simulink subsystem "Trayectoria"  (R2024b)
settings: Solver=VariableStepAuto  StartTime=0.0  StopTime=10.0  RelTol=1e-3
libraries: slpidlib x1
settings Model: Creator=Chenfu  LastModifiedBy=Chenfu

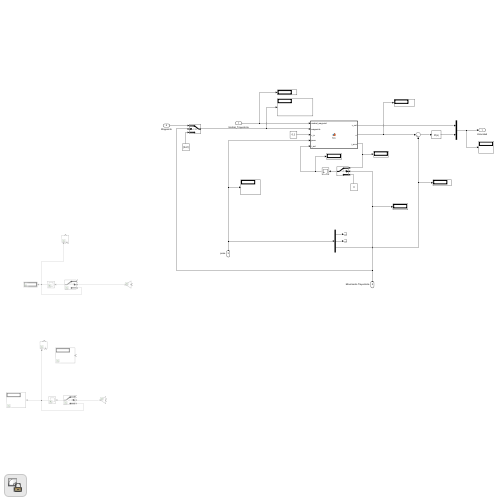
[thumbnail: Simulink's stored preview of the top-level diagram]
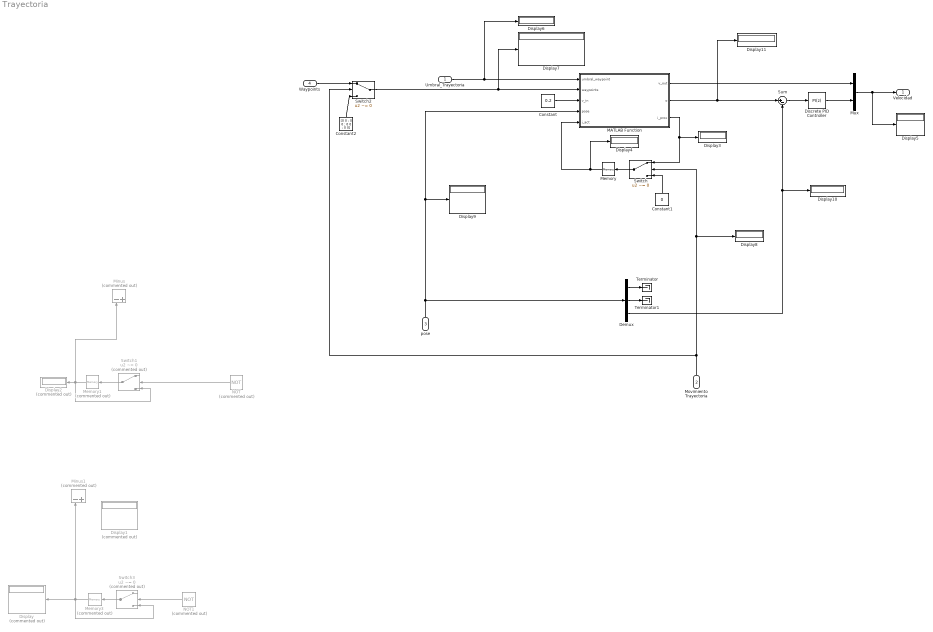
== system Trayectoria ==
  Umbral_Trayectoria : Inport
  Movimiento Trayectoria : Inport  Port=2
  pose : Inport  Port=3
  Waypoints : Inport  Port=4
  Constant : Constant  Value=0.2
  Constant1 : Constant  Value=0
  Constant2 : Constant  Value=[0 0 ; 0 0 ; 0 0 ; 0 0]
  Demux : Demux  Outputs=3
  Discrete PID Controller : slpidlib/PID Controller  Controller=PI  Form=Parallel  TimeDomain=Discrete-time  UseExternalTs=off  SampleTime=0.01  IntegratorMethod=Forward Euler  FilterMethod=Forward Euler  ControllerParametersSource=internal  P=0.909134313735057  I=0.0143713686377566  UseKiTs=off  D=0  UseExternalDerivativeSource=off  N=100  UseFilter=on  TunerSelectOption=Transfer Function Based (PID Tuner App)  InitialConditionSource=internal  InitialConditionForIntegrator=0  InitialConditionForFilter=0  DifferentiatorICPrevScaledInput=0  ExternalReset=none  TrackingMode=off  Kt=1  LimitOutput=off  SatLimitsSource=internal  UpperSaturationLimit=inf  LowerSaturationLimit=-inf  LinearizeAsGain=off  AntiWindupMode=none  Kb=1  LimitIntegrator=off  UpperIntegratorSaturationLimit=inf  LowerIntegratorSaturationLimit=-inf  POutMin=[]  POutMax=[]  IOutMin=[]  IOutMax=[]  DOutMin=[]  DOutMax=[]  NOutMin=[]  NOutMax=[]  SumOutMin=[]  SumOutMax=[]  SaturationOutMin=[]  SaturationOutMax=[]  PParamMin=[]  PParamMax=[]  IParamMin=[]  IParamMax=[]  DParamMin=[]  DParamMax=[]  NParamMin=[]  NParamMax=[]  KbParamMin=[]  KbParamMax=[]  KtParamMin=[]  KtParamMax=[]  KbOutMin=[]  KbOutMax=[]  KtOutMin=[]  KtOutMax=[]  IntegratorOutMin=[]  IntegratorOutMax=[]  FilterOutMin=[]  FilterOutMax=[]  SumI1OutMin=[]  SumI1OutMax=[]  SumI2OutMin=[]  SumI2OutMax=[]  SumI3OutMin=[]  SumI3OutMax=[]  SumI4OutMin=[]  SumI4OutMax=[]  SumDOutMin=[]  SumDOutMax=[]  DifferentiatorOutMin=[]  DifferentiatorOutMax=[]  FilterDiffOutCoefMin=[]  FilterDiffOutCoefMax=[]  ReciprocalOutMin=[]  ReciprocalOutMax=[]  SumDenOutMin=[]  SumDenOutMax=[]  SumNumOutMin=[]  SumNumOutMax=[]  DivideOutMin=[]  DivideOutMax=[]  UdiffTsProdOutMin=[]  UdiffTsProdOutMax=[]  NTsProdOutMin=[]  NTsProdOutMax=[]  UintegralTsProdOutMin=[]  UintegralTsProdOutMax=[]  UngainTsProdOutMin=[]  UngainTsProdOutMax=[]  ClampingZeroOutDataTypeStr=Inherit: Inherit via back propagation  ClampingZeroOutMin=[]  ClampingZeroOutMax=[]  FilterDenConstantOutDataTypeStr=Inherit: Inherit via back propagation  FilterDenConstantOutMin=[]  FilterDenConstantOutMax=[]  PCopyOutDataTypeStr=Inherit: Inherit via back propagation  PCopyOutMin=[]  PCopyOutMax=[]  NCopyOutDataTypeStr=Inherit: Inherit via back propagation  NCopyOutMin=[]  NCopyOutMax=[]  IntegratorContinuousStateAttributes=''  IntegratorStateMustResolveToSignalObject=off  IntegratorRTWStateStorageClass=Auto  FilterContinuousStateAttributes=''  FilterStateMustResolveToSignalObject=off  FilterRTWStateStorageClass=Auto  ParallelPVariant=InternalParameters  IdealPVariant=Disabled  IVariant=InternalParameters  DVariant=Disabled  IntegratorVariant=Discrete  SatVariant=Disabled  AWVariant=Passthrough  PCopyVariant=Disabled  TRVariant=Disabled  FdbkBlocksVariant=Forward  IdealPFdbkVariant=Disabled  SatFdbkVariant=Disabled  DerivativeFilterVariant=Disabled  NVariant=Disabled  NCopyVariant=Disabled_SignalSpec  FilterICVariant=Disabled  IntegratorICVariant=InternalICs  ExternalResetVariant=Disabled  TRSumVariant=Passthrough  SumFdbkVariant=Disabled  SumVariant=Sum_PI  TsampFilterVariant=InternalTs  TsampNgainVariant=Passthrough  TsampIntegralVariant=Disabled_SignalSpec  ExternalSaturationOutDataTypeStr=Inherit: Same as second input  DerivativeSourceVariant=Disabled  PreIntVariant=InternalPreInt
      settings: LibrarySourceBlock=simulink/Discrete/Discrete PID Controller
  Display : Display  Commented=on
  Display1 : Display  Commented=on
  Display{3..11} (9 alike) : Display
  Display2 : Display  Commented=on
  MATLAB Function : MATLAB Function  TreatAsAtomicUnit=on
  Memory : Memory
  Memory1 : Memory  Commented=on
  Memory3 : Memory  Commented=on
  Minus : Sum  Commented=on  Inputs=-+
  Minus1 : Sum  Commented=on  Inputs=-+
  Mux : Mux  Inputs=2
  NOT : Logic  Commented=on  Operator=NOT  IconShape=distinctive  AllPortsSameDT=off  OutDataTypeStr=boolean
  NOT1 : Logic  Commented=on  Operator=NOT  IconShape=distinctive  AllPortsSameDT=off  OutDataTypeStr=boolean
  Sum : Sum  Inputs=|+-
  Switch : Switch  Criteria=u2 ~= 0  SaturateOnIntegerOverflow=off  InputSameDT=off
  Switch1 : Switch  Commented=on  Criteria=u2 ~= 0  SaturateOnIntegerOverflow=off  InputSameDT=off
  Switch2 : Switch  Criteria=u2 ~= 0  SaturateOnIntegerOverflow=off  InputSameDT=off
  Switch3 : Switch  Commented=on  Criteria=u2 ~= 0  SaturateOnIntegerOverflow=off  InputSameDT=off
  Terminator : Terminator
  Terminator1 : Terminator
  Velocidad : Outport
  wires:
  Sum/1 -> Discrete PID Controller/1
  Constant/1 -> MATLAB Function/3(v_in)
  MATLAB Function/2(o) -> Sum/1, Display11/1
  Demux/1 -> Terminator/1
  Demux/2 -> Terminator1/1
  Demux/3 -> Display10/1, Sum/2
  Switch2/1 -> MATLAB Function/2(waypoints), Display7/1
  MATLAB Function/1(v_out) -> Mux/1
  Discrete PID Controller/1 -> Mux/2
  Mux/1 -> Velocidad/1, Display5/1
  Switch/1 -> Memory/1
  MATLAB Function/3(i_prox) -> Display3/1, Switch/1
  Movimiento Trayectoria/1 -> Switch/2, Display8/1, Switch2/2
  Memory/1 -> Display4/1, MATLAB Function/5(i_act)
  pose/1 -> Demux/1, Display9/1, MATLAB Function/4(pose)
  Umbral_Trayectoria/1 -> MATLAB Function/1(umbral_waypoint), Display6/1
  Constant1/1 -> Switch/3
  Memory1/1 -> Switch1/3, Display2/1, Minus/1
  Switch1/1 -> Memory1/1
  NOT/1 -> Switch1/2
  Memory3/1 -> Minus1/1, Display/1, Switch3/3
  Switch3/1 -> Memory3/1
  NOT1/1 -> Switch3/2
  Waypoints/1 -> Switch2/1
  Constant2/1 -> Switch2/3

== matlab function Trayectoria/MATLAB Function ==
  data: umbral_waypoint input; waypoints input; v_in input; v_out output size=1; o output size=1; pose input; i_act input; i_prox output size=1
function [v_out,o,i_prox] = fcn(umbral_waypoint,waypoints,v_in,pose,i_act)

i_prox = i_act + 1;

x_pose = pose(1);
y_pose = pose(2);

% Si sigue habiendo waypoints -> Se mueve
if(size(waypoints,1) >= i_prox)
    x_waypoint = waypoints(i_prox,1);
    y_waypoint = waypoints(i_prox,2);

    dist = sqrt((x_waypoint-x_pose)^2+(y_waypoint-y_pose)^2);
    
    % Si está lejos de waypoint -> Sigue yendo al mismo waypoint
    if (dist > umbral_waypoint)
       i_prox = i_prox - 1;
    end
v_out = v_in;
o = atan2(y_waypoint-y_pose,x_waypoint-x_pose);

% Si ya no hay mas waypoints -> se para el robot.
else

v_out = 0;
o = 0;
i_prox = i_act;

end
